simulink model "ParameterizeMotorTorque"  (R2023b)
settings: Solver=VariableStepAuto  StartTime=0.0  StopTime=10  RelTol=1e-3  EnableMultiTasking=on
PreLoadFcn:
  | load ParameterizeMotorTorqueData
  | x0 = 20;
  | xmin = 20;
  | xmax = 70;
  | V = 13.5;
values from neighbouring files (symbols this model uses):
  ni = 13    [ParameterizeMotorTorqueData.mat]
  nx = 46    [ParameterizeMotorTorqueData.mat]
libraries: fl_lib x20, nesl_utility x7, ee_lib x3
CloseFcn:
  | try,close(h1_ParameterizeMotorTorque),end
  | clear h1_ParameterizeMotorTorque
  | try,close(h2_ParameterizeMotorTorque),end
  | clear h2_ParameterizeMotorTorque
  | try,close(h3_ParameterizeMotorTorque),end
  | clear h3_ParameterizeMotorTorque
  | try,close(h4_ParameterizeMotorTorque),end
  | clear h4_ParameterizeMotorTorque
  | try,close(h5_ParameterizeMotorTorque),end
  | clear h5_ParameterizeMotorTorque
  | 
  | clear simlog_ParameterizeMotorTorque
  | clear logsout_ParameterizeMotorTorque
  | clear TorqueData V angle current d2r data dfluxdx i nAngPts nCurrPts ni nx p r2d temp_colororder torque tout trq trq0A trq1A trq2A trq3A trq4A trq5A trq6A trqData v x x0 xmax xmin
Description:
  | Torque Motor Parameterization
settings Model: FPTRunName=Active  Creator=The MathWorks, Inc.  LastModifiedBy=simon
settings SolverCC: AlgebraicLoopSolver=TrustRegion
settings DataIOCC: LimitDataPoints=on  MaxDataPoints=10000  SaveFormat=Array  ReturnWorkspaceOutputs=off  SignalLoggingName=logsout_ParameterizeMotorTorque
settings OptimizationCC: ReuseModelBlockBuffer=off  ExpressionDepthLimit=2147483647  InitFltsAndDblsToZero=on  LifeSpan=inf
settings DebuggingCC: UnderspecifiedInitializationDetection=Classic  MergeDetectMultiDrivingBlocksExec=none  FcnCallInpInsideContextMsg=warning  UnconnectedInputMsg=warning  UnconnectedOutputMsg=warning  UnconnectedLineMsg=warning  AllowSymbolicDim=off  StateNameClashWarn=warning  SFUnexpectedBacktrackingDiag=warning  SFNoUnconditionalDefaultTransitionDiag=warning  SFExecutionAtInitializationDiag=none  ArithmeticOperatorsInVariantConditions=warning
settings HardwareCC: ProdBitPerPointer=32  ProdBitPerSizeT=32  ProdBitPerPtrDiffT=32  ProdLargestAtomicFloat=None  ProdIntDivRoundTo=Undefined  ProdEndianess=Unspecified  ProdWordSize=32  ProdHWDeviceType=32-bit Generic
settings ModelReferenceCC: EnableRefExpFcnMdlSchedulingChecks=on  PropagateSignalLabelsOutOfModel=off
settings SFSimCC: SimUseLocalCustomCode=off  CustomCodeUndefinedFunction=UseInterfaceOnly
settings RTWCC: RTWUseLocalCustomCode=off  DLArmComputeVersion=19.05
settings CodeAppCC: StateflowObjectComments=on
settings GRTTargetCC: TargetLangStandard=C89/C90 (ANSI)  CombineOutputUpdateFcns=off  GRTInterface=on
settings ConfigComp: CovMetricSettings=dw  CovSaveCumulativeToWorkspaceVar=on  CovSaveSingleToWorkspaceVar=on  CovExternalEMLEnable=off  CovSFcnEnable=off
settings SimscapeCC: SimscapeLogType=all  SimscapeLogSimulationStatistics=on  SimscapeLogName=simlog_ParameterizeMotorTorque  SimscapeLogDataHistory=10000

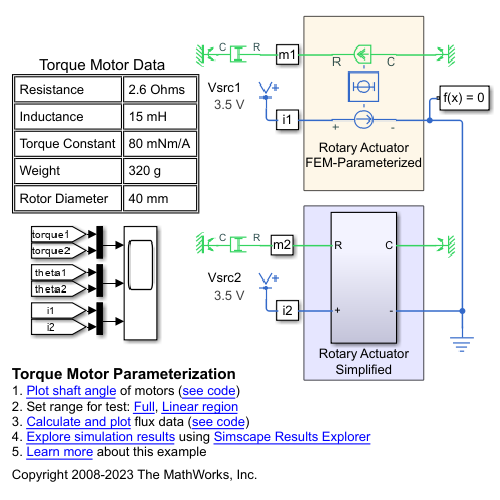
[thumbnail: Simulink's stored preview of the top-level diagram]
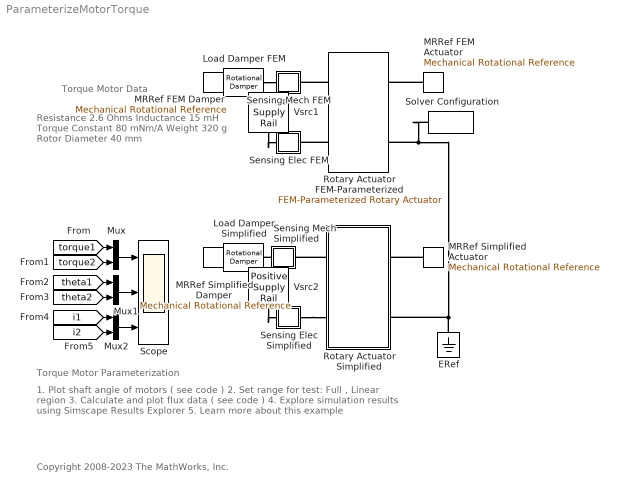
== system ParameterizeMotorTorque ==
  note: Torque Motor Data
  note: Resistance
      | 2.6 Ohms
      |
      | Inductance
      | 15 mH
      |
      | Torque Constant
      | 80 mNm/A
      |
      | Weight
      | 320 g
      |
      | Rotor Diameter
      | 40 mm
  note: Torque Motor Parameterization
  note: 1. Plot shaft angle of motors ( see code )
      | 2. Set range for test: Full , Linear region
      | 3. Calculate and plot flux data ( see code )
      | 4. Explore simulation results using Simscape Results Explorer
      | 5. Learn more about this example
  note: Copyright 2008-2023 The MathWorks, Inc.
  ERef : fl_lib/Electrical/Electrical Elements/Electrical Reference
  Load Damper FEM : fl_lib/Mechanical/Rotational Elements/Rotational Damper  D=1 N*m/(rad/s)  w_specify=off  w_priority=High  w=0 rad/s  w_nominal_specify=off  w_nominal_unit=rad/s  w_nominal_value=1  t_specify=off  t_priority=High  t=0 N*m  t_nominal_specify=off  t_nominal_unit=N*m  t_nominal_value=1
  Load Damper Simplified : fl_lib/Mechanical/Rotational Elements/Rotational Damper  D=1 N*m/(rad/s)  w_specify=off  w_priority=High  w=0 rad/s  w_nominal_specify=off  w_nominal_unit=rad/s  w_nominal_value=1  t_specify=off  t_priority=High  t=0 N*m  t_nominal_specify=off  t_nominal_unit=N*m  t_nominal_value=1
  MRRef FEM Actuator : fl_lib/Mechanical/Rotational Elements/Mechanical Rotational Reference
  MRRef FEM Damper : fl_lib/Mechanical/Rotational Elements/Mechanical Rotational Reference
  MRRef Simplified Actuator : fl_lib/Mechanical/Rotational Elements/Mechanical Rotational Reference
  MRRef Simplified Damper : fl_lib/Mechanical/Rotational Elements/Mechanical Rotational Reference
  Mux : Mux  Inputs=2
  Mux1 : Mux  Inputs=2
  Mux2 : Mux  Inputs=2
  "Rotary Actuator FEM-Parameterized " : ee_lib/Electromechanical/Mechatronic Actuators/FEM-Parameterized Rotary Actuator  src_type=2  iVec=current A  xVec=x rad  dfluxdiMatrix=15e-3*ones(ni,nx) Wb/A  dfluxdxMatrix=dfluxdx Wb/rad  FluxMatrix=[ 0 0 0 0 0 0 0 0 0 0 0 0 0 0 0 0 0 0 0; 4e-4 4.8e-4 7e-4 0.00105 0.00147 0.00193 0.00235 0.0027 0.00292 0.003 0.00292 0.0027 0.00235 0.00193 0.00147 0.00105 7e-4 4.8e-4 4e-4; 8e-4 9.6e-4 0.00141 0.0021 0.00295 0.00385 0.0047 0.00539 0.00584 0.006 0.00584 0.00539 0.0047 0.00385 0.00295 0.0021 0.00141 9.6e-4 8e-4; 0.0012 0.00144 0.00211 0.00315 0.00442 0.00578 0.00705 0.00809 0.00876 0.008999999999999999 0.00876 0.00809 0.00705 0.00578 0.00442 0.00315 0.00211 0.00144 0.0012; 0.0016 0.00191 0.00282 0.0042 0.0059 0.0077 0.0094 0.01078 0.01169 0.012 0.01169 0.01078 0.0094 0.0077 0.0059 0.0042 0.00282 0.00191 0.0016; 0.002 0.00239 0.00352 0.00525 0.00737 0.00963 0.01175 0.01348 0.01461 0.015 0.01461 0.01348 0.01175 0.00963 0.00737 0.00525 0.00352 0.00239 0.002 ] Wb  calculate_torque_matrix=0  TorqueMatrix=torque N*m  cyclic=1  interp_method=1  extrap_method=1  R1=2.6 Ohm  Rm=inf Ohm  lam=0 N*m/(rad/s)  Inertia=200 g*cm^2  Xmin=xmin deg  Xmax=xmax deg  K_endstop=1e+7 N*m/rad  D_endstop=100 N*m/(rad/s)  i_specify=off  i_priority=None  i=0 A  i_nominal_specify=off  i_nominal_unit=A  i_nominal_value=1  Trq_specify=off  Trq_priority=None  Trq=0 N*m  Trq_nominal_specify=off  Trq_nominal_unit=N*m  Trq_nominal_value=1  x_specify=on  x_priority=High  x=x0 deg  x_nominal_specify=off  x_nominal_unit=deg  x_nominal_value=1  w_specify=on  w_priority=Low  w=0 deg/s  w_nominal_specify=off  w_nominal_unit=deg/s  w_nominal_value=1  magnetic_torque_specify=off  magnetic_torque_priority=None  magnetic_torque=0 N*m  magnetic_torque_nominal_specify=off  magnetic_torque_nominal_unit=N*m  magnetic_torque_nominal_value=1  alpha=3.93e-3 1/K  Tmeas=25 degC  thermal_mass=100 J/K  T_specify=off  T_priority=High  T=300 K  T_nominal_specify=off  T_nominal_unit=K  T_nominal_value=1
      settings: InternalSimscapePortConfiguration="{\"Bottom\":[],\"Left\":[{\"id\":\"p\",\"label\":\"+\",\"type\":\"foundation.electrical.electrical\"},{\"id\":\"R\",\"label\":\"R\",\"type\":\"foundation.mechanical.rotational.rotational\"}],\"Right\":[{\"id\":\"n\",\"label\":\"-\",\"type\":\"foundation.electrical.electrical\"},{\"id\":\"C\",\"label\":\"C\",\"type\":\"foundation.mechanical.rotational.rotational\"}],\"Top\":[]}"
  "Rotary Actuator Simplified " : Subsystem  Tag=PublishSubsystem
  Scope : Scope  NumInputPorts=3
  Sensing Elec FEM : Subsystem
      mask Display: disp('i1');
  Sensing Elec Simplified : Subsystem
      mask Display: disp('i2');
  "Sensing Mech FEM " : Subsystem
      mask Display: disp('m1')
  Sensing Mech Simplified : Subsystem
      mask Display: disp('m2')
  Solver Configuration : nesl_utility/Solver Configuration  PhysicalDomain=network_engine_domain  SubClassName=solver  LeftPortType=input  RightPortType=generic  Tones=[]  Harmonics=[]  SimulateNoise=off  Profile=off  UseLocalSampling=off  EnableSwitchedLinearOptims=on  FrequencyDomain=off  UseCCode=off  RelTol=0.001  AbsTol=1e-06  MinStep=1e-09  ToWorkspace=off  RevertToSquareIcSolve=off  NumHomotopyIterations=100  PhasorMode=off  PhasorModeNumHarmonics=1  ConsistencySolver=NEWTON_FTOL  IndexReductionMethod=DerivativeReplacement  DoDC=off  ResidualTolerance=1e-9  ConsistencyTolSource=GLOBAL  ConsistencyAbsTol=0.001  ConsistencyRelTol=0.001  ConsistencyTolFactor=0.001  UseLocalSolver=off  LocalSolverChoice=NE_BACKWARD_EULER_ADVANCER  ResolveIndetEquations=on  FunctionEvalNumThread=1  LocalSolverSampleTime=.001  DoFixedCost=off  MaxNonlinIter=3  MaxModeIter=2  ComputeImpulses=off  ImpulseIterations=2  LinearAlgebra=auto  LinearAlgebraNumThread=0  EquationFormulation=NE_TIME_EF  DelaysMemoryBudget=1024  AutomaticFiltering=on  FilteringTimeConstant=0.001  PartitionStorageMethod=AS_NEEDED  PartitionMemoryBudget=1024  PartitionMethod=FAST  MultibodyUseLocalSolver=off  MultibodyLocalSolverChoice=ODE1  MultibodyLocalSolverSampleTime=0.001
  Vsrc1 : ee_lib/Sources/Positive Supply Rail  v0=3.5 V
      settings: AttributesFormatString=%<v0> %<v0_unit>  InternalSimscapePortConfiguration="{\"Bottom\":[],\"Left\":[],\"Right\":[{\"id\":\"p\",\"label\":\"\",\"type\":\"foundation.electrical.electrical\"}],\"Top\":[]}"
  Vsrc2 : ee_lib/Sources/Positive Supply Rail  v0=3.5 V
      settings: AttributesFormatString=%<v0> %<v0_unit>  InternalSimscapePortConfiguration="{\"Bottom\":[],\"Left\":[],\"Right\":[{\"id\":\"p\",\"label\":\"\",\"type\":\"foundation.electrical.electrical\"}],\"Top\":[]}"
  wires:
  [torque1] -> Mux/1
  [torque2] -> Mux/2
  Mux/1 -> Scope/1
  [theta1] -> Mux1/1
  [theta2] -> Mux1/2
  Mux1/1 -> Scope/2
  [i1] -> Mux2/1
  [i2] -> Mux2/2
  Mux2/1 -> Scope/3
  connections:
  ERef/LConn1 -- Solver Configuration/RConn1 -- "Rotary Actuator FEM-Parameterized "/RConn1 -- "Rotary Actuator Simplified "/RConn2
  Load Damper FEM/LConn1 -- "Sensing Mech FEM "/RConn1
  Sensing Mech Simplified/RConn1 -- Load Damper Simplified/LConn1
  "Rotary Actuator FEM-Parameterized "/LConn2 -- "Sensing Mech FEM "/LConn1
  "Rotary Actuator FEM-Parameterized "/LConn1 -- Sensing Elec FEM/RConn1
  MRRef FEM Actuator/LConn1 -- "Rotary Actuator FEM-Parameterized "/RConn2
  "Rotary Actuator Simplified "/LConn1 -- Sensing Mech Simplified/LConn1
  Sensing Elec Simplified/RConn1 -- "Rotary Actuator Simplified "/LConn2
  Load Damper FEM/RConn1 -- MRRef FEM Damper/LConn1
  MRRef Simplified Damper/LConn1 -- Load Damper Simplified/RConn1
  Vsrc1/RConn1 -- Sensing Elec FEM/LConn1
  Vsrc2/RConn1 -- Sensing Elec Simplified/LConn1
  MRRef Simplified Actuator/LConn1 -- "Rotary Actuator Simplified "/RConn1

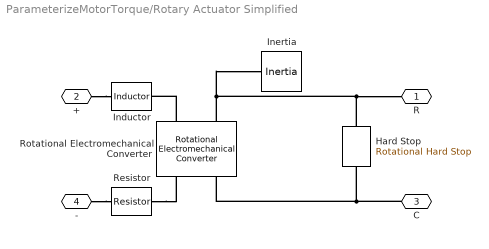
== system ParameterizeMotorTorque/Rotary Actuator Simplified  ==
  Hard Stop : fl_lib/Mechanical/Rotational Elements/Rotational Hard Stop  upper_bnd=xmax deg  lower_bnd=xmin deg  model=3  stiff_up=1e+7 N*m/rad  stiff_low=1e+7 N*m/rad  D_up=100 N*m/(rad/s)  D_low=100 N*m/(rad/s)  transition=0.001 rad  coeff_rest=0.7  w_tol=0.1 rad/s  trq_tol=0.001 N*m  w_specify=off  w_priority=High  w=0 rad/s  w_nominal_specify=off  w_nominal_unit=rad/s  w_nominal_value=1  t_specify=off  t_priority=High  t=0 N*m  t_nominal_specify=off  t_nominal_unit=N*m  t_nominal_value=1  phi_specify=on  phi_priority=High  phi=x0 deg  phi_nominal_specify=off  phi_nominal_unit=rad  phi_nominal_value=1  M_specify=off  M_priority=None  M=0
  Inductor : fl_lib/Electrical/Electrical Elements/Inductor  l=15 mH  r=0 Ohm  g=1e-9 1/Ohm  i_specify=off  i_priority=High  i=0 A  i_nominal_specify=off  i_nominal_unit=A  i_nominal_value=1  v_specify=off  v_priority=High  v=0 V  v_nominal_specify=off  v_nominal_unit=V  v_nominal_value=1  i_L_specify=on  i_L_priority=High  i_L=0 A  i_L_nominal_specify=off  i_L_nominal_unit=A  i_L_nominal_value=1
  Inertia : fl_lib/Mechanical/Rotational Elements/Inertia  inertia=200 g*cm^2  num_ports=foundation.enum.numPorts2.one  w_specify=on  w_priority=High  w=0 rad/s  w_nominal_specify=off  w_nominal_unit=rad/s  w_nominal_value=1  t_specify=off  t_priority=High  t=0 N*m  t_nominal_specify=off  t_nominal_unit=N*m  t_nominal_value=1
  Resistor : fl_lib/Electrical/Electrical Elements/Resistor  R=2.6 Ohm  i_specify=off  i_priority=High  i=0 A  i_nominal_specify=off  i_nominal_unit=A  i_nominal_value=1  v_specify=off  v_priority=High  v=0 V  v_nominal_specify=off  v_nominal_unit=V  v_nominal_value=1
  Rotational Electromechanical Converter : fl_lib/Electrical/Electrical Elements/Rotational Electromechanical Converter  K=80e-3 V/(rad/s)  i_specify=off  i_priority=High  i=0 A  i_nominal_specify=off  i_nominal_unit=A  i_nominal_value=1  v_specify=off  v_priority=High  v=0 V  v_nominal_specify=off  v_nominal_unit=V  v_nominal_value=1  t_specify=off  t_priority=High  t=0 N*m  t_nominal_specify=off  t_nominal_unit=N*m  t_nominal_value=1  w_specify=off  w_priority=High  w=0 rad/s  w_nominal_specify=off  w_nominal_unit=rad/s  w_nominal_value=1
  R : PMIOPort  Side=Left
  + : PMIOPort  Port=2  Side=Left
  C : PMIOPort  Port=3  Side=Right
  - : PMIOPort  Port=4  Side=Right
  connections:
  +/RConn1 -- Inductor/LConn1
  C/RConn1 -- Rotational Electromechanical Converter/RConn2 -- Hard Stop/RConn1
  -/RConn1 -- Resistor/LConn1
  Resistor/RConn1 -- Rotational Electromechanical Converter/RConn1
  Rotational Electromechanical Converter/LConn1 -- Inductor/RConn1
  Hard Stop/LConn1 -- R/RConn1 -- Rotational Electromechanical Converter/LConn2 -- Inertia/LConn1

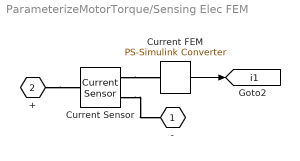
== system ParameterizeMotorTorque/Sensing Elec FEM ==
  Current Sensor : fl_lib/Electrical/Electrical Sensors/Current Sensor
  Current FEM : nesl_utility/PS-Simulink Converter  PhysicalDomain=network_engine_domain  SubClassName=ps_output  LeftPortType=input  RightPortType=output  PseudoPeriodic=off  Frequencies=[]  VectorFormat=1-D array  Unit=A  AffineConversion=off
  - : PMIOPort  Side=Right
  + : PMIOPort  Port=2  Side=Left
  tag scope: i1=global
  wires:
  Current FEM/1 -> [i1]
  connections:
  Current Sensor/RConn1 -- Current FEM/LConn1
  Current Sensor/RConn2 -- -/RConn1
  +/RConn1 -- Current Sensor/LConn1

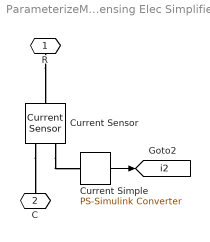
== system ParameterizeMotorTorque/Sensing Elec Simplified ==
  Current Sensor : fl_lib/Electrical/Electrical Sensors/Current Sensor
  Current Simple : nesl_utility/PS-Simulink Converter  PhysicalDomain=network_engine_domain  SubClassName=ps_output  LeftPortType=input  RightPortType=output  PseudoPeriodic=off  Frequencies=[]  VectorFormat=1-D array  Unit=A  AffineConversion=off
  R : PMIOPort  Side=Left
  C : PMIOPort  Port=2  Side=Right
  tag scope: i2=global
  wires:
  Current Simple/1 -> [i2]
  connections:
  R/RConn1 -- Current Sensor/LConn1
  Current Sensor/RConn2 -- C/RConn1
  Current Sensor/RConn1 -- Current Simple/LConn1

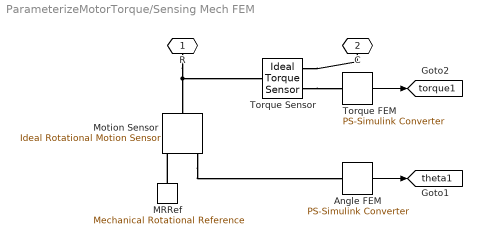
== system ParameterizeMotorTorque/Sensing Mech FEM  ==
  Angle FEM : nesl_utility/PS-Simulink Converter  PhysicalDomain=network_engine_domain  SubClassName=ps_output  LeftPortType=input  RightPortType=output  PseudoPeriodic=off  Frequencies=[]  VectorFormat=1-D array  Unit=deg  AffineConversion=off
  MRRef : fl_lib/Mechanical/Rotational Elements/Mechanical Rotational Reference
  Motion Sensor : fl_lib/Mechanical/Mechanical Sensors/Ideal Rotational Motion Sensor  reference=foundation.enum.MeasurementReference.difference  acceleration_port=false  velocity_port=true  position_port=true  wrap_angle=simscape.enum.onoff.off  offset=x0 deg
  Torque FEM : nesl_utility/PS-Simulink Converter  PhysicalDomain=network_engine_domain  SubClassName=ps_output  LeftPortType=input  RightPortType=output  PseudoPeriodic=off  Frequencies=[]  VectorFormat=1-D array  Unit=N*m  AffineConversion=off
  Torque Sensor : fl_lib/Mechanical/Mechanical Sensors/Ideal Torque Sensor
  R : PMIOPort  Side=Left
  C : PMIOPort  Port=2  Side=Right
  tag scope: theta1=global, torque1=global
  wires:
  Angle FEM/1 -> [theta1]
  Torque FEM/1 -> [torque1]
  connections:
  Torque Sensor/RConn2 -- Torque FEM/LConn1
  Motion Sensor/RConn3 -- Angle FEM/LConn1
  Torque Sensor/RConn1 -- C/RConn1
  R/RConn1 -- Torque Sensor/LConn1 -- Motion Sensor/LConn1
  MRRef/LConn1 -- Motion Sensor/RConn1

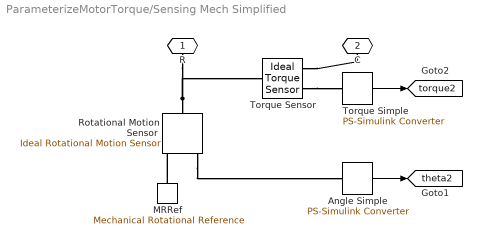
== system ParameterizeMotorTorque/Sensing Mech Simplified ==
  Angle Simple : nesl_utility/PS-Simulink Converter  PhysicalDomain=network_engine_domain  SubClassName=ps_output  LeftPortType=input  RightPortType=output  PseudoPeriodic=off  Frequencies=[]  VectorFormat=1-D array  Unit=deg  AffineConversion=off
  MRRef : fl_lib/Mechanical/Rotational Elements/Mechanical Rotational Reference
  Rotational Motion Sensor : fl_lib/Mechanical/Mechanical Sensors/Ideal Rotational Motion Sensor  reference=foundation.enum.MeasurementReference.difference  acceleration_port=false  velocity_port=true  position_port=true  wrap_angle=simscape.enum.onoff.off  offset=x0 deg
  Torque Sensor : fl_lib/Mechanical/Mechanical Sensors/Ideal Torque Sensor
  Torque Simple : nesl_utility/PS-Simulink Converter  PhysicalDomain=network_engine_domain  SubClassName=ps_output  LeftPortType=input  RightPortType=output  PseudoPeriodic=off  Frequencies=[]  VectorFormat=1-D array  Unit=N*m  AffineConversion=off
  R : PMIOPort  Side=Left
  C : PMIOPort  Port=2  Side=Right
  tag scope: theta2=global, torque2=global
  wires:
  Torque Simple/1 -> [torque2]
  Angle Simple/1 -> [theta2]
  connections:
  MRRef/LConn1 -- Rotational Motion Sensor/RConn1
  Rotational Motion Sensor/LConn1 -- Torque Sensor/LConn1 -- R/RConn1
  Torque Sensor/RConn1 -- C/RConn1
  Rotational Motion Sensor/RConn3 -- Angle Simple/LConn1
  Torque Sensor/RConn2 -- Torque Simple/LConn1
